simulink library "MinSegLibrary_M2V5"  (R2015a)
settings: Solver=ode45  StartTime=0.0  StopTime=10.0  RelTol=1e-3
libraries: arduinolib x8
settings Model: Creator=hurstj  LastModifiedBy=hurstj
settings DebuggingCC: UnderspecifiedInitializationDetection=Classic  MergeDetectMultiDrivingBlocksExec=none  SolverPrmCheckMsg=warning  StateNameClashWarn=warning

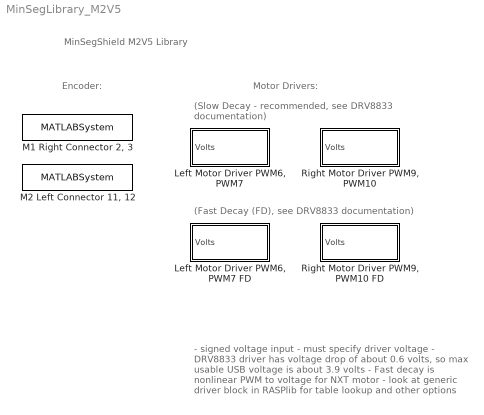
== system MinSegLibrary_M2V5 ==
  note: Encoder:
  note: MinSegShield M2V5 Library
  note: (Slow Decay - recommended, see DRV8833 documentation)
  note: Motor Drivers:
  note: (Fast Decay (FD), see DRV8833 documentation)
  note: - signed voltage input
      | - must specify driver voltage
      | - DRV8833 driver has voltage drop of about 0.6 volts, so max usable USB voltage is about 3.9 volts
      | - Fast decay is nonlinear PWM to voltage for NXT motor
      | - look at generic driver block in RASPlib for table lookup and other options
  "Left Motor Driver PWM6, PWM7" : Subsystem  mask{Vsupply=3.9, PWMoffset=0}
      mask prompts: Vsupply "Driver Voltage"; PWMoffset "PWM offset (0-255)"
      mask help:
      | Specify driver supply voltage (3.9 for USB)
      | Specify the PWM offset (0-255)
      mask Display:
      | port_label('input',1,'Volts')
      | text(15,5,['Vsupply=' num2str(Vsupply)])
  "Left Motor Driver PWM6, PWM7 FD" : Subsystem  mask{Vsupply=3.9, PWMoffset=0}
      mask prompts: Vsupply "Driver Voltage"; PWMoffset "PWM offset (0-255)"
      mask help:
      | Specify driver supply voltage (3.9 for USB)
      | Specify the PWM offset (0-255)
      mask Display:
      | port_label('input',1,'Volts')
      | text(15,5,['Vsupply=' num2str(Vsupply)])
  "M1 Right Connector 2, 3" : MATLABSystem  System=Encoder_arduino  Encoder=0  PinA=2  PinB=3
      mask Type: Encoder_arduino
      mask Display:
      | disp('soEncoder');
      | port_label('output',1,'y');
  "M2 Left Connector 11, 12" : MATLABSystem  System=Encoder_arduino  Encoder=4  PinA=11  PinB=12
      mask Type: Encoder_arduino
      mask Display:
      | disp('soEncoder');
      | port_label('output',1,'y');
  "Right Motor Driver PWM9, PWM10 " : Subsystem  mask{Vsupply=3.9, PWMoffset=0}
      mask prompts: Vsupply "Driver Voltage"; PWMoffset "PWM offset (0-255)"
      mask help:
      | Specify driver supply voltage (3.9 for USB)
      | Specify the PWM offset (0-255)
      mask Display:
      | port_label('input',1,'Volts')
      | text(15,5,['Vsupply=' num2str(Vsupply)])
  "Right Motor Driver PWM9, PWM10 FD" : Subsystem  mask{Vsupply=3.9, PWMoffset=0}
      mask prompts: Vsupply "Driver Voltage"; PWMoffset "PWM offset (0-255)"
      mask help:
      | Specify driver supply voltage (3.9 for USB)
      | Specify the PWM offset (0-255)
      mask Display:
      | port_label('input',1,'Volts')
      | text(15,5,['Vsupply=' num2str(Vsupply)])

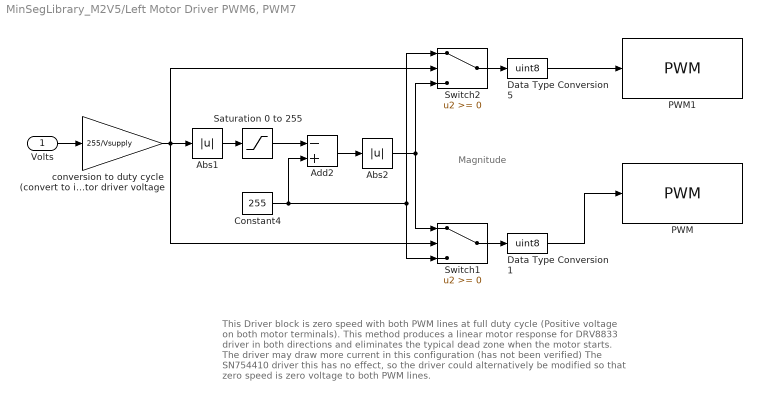
== system MinSegLibrary_M2V5/Left Motor Driver PWM6, PWM7 ==
  note: This Driver block is zero speed with both PWM lines at full duty cycle
      |  (Positive voltage on both motor terminals).
      | This method produces a linear motor response for DRV8833 driver
      |  in both directions and eliminates
      | the typical dead zone when the motor starts.
      | The driver may draw more current in this configuration (has not been verified)
      |
      | The SN754410 driver this has no effect, so the driver could alternatively
      | be modified so that zero speed is zero voltage to both PWM lines.
  note: Magnitude
  Volts : Inport
  Abs1 : Abs
  Abs2 : Abs
  Add2 : Sum  Inputs=-+
  Constant4 : Constant  Value=255
  Data Type Conversion1 : DataTypeConversion  OutDataTypeStr=uint8
  Data Type Conversion5 : DataTypeConversion  OutDataTypeStr=uint8
  PWM : arduinolib/PWM  pinNumber=7  blockPlatform=arduino
  PWM1 : arduinolib/PWM  pinNumber=6  blockPlatform=arduino
  Saturation 0 to 255 : Saturate  UpperLimit=255  LowerLimit=0
  Switch1 : Switch
  Switch2 : Switch
  conversion to duty cycle (convert to int) denominator is motor driver voltage : Gain  Gain=255/Vsupply  OutDataTypeStr=int16
  wires:
  Volts/1 -> conversion to duty cycle (convert to int) denominator is motor driver voltage/1
  conversion to duty cycle (convert to int) denominator is motor driver voltage/1 -> Switch2/2, Abs1/1, Switch1/2
  Saturation 0 to 255/1 -> Add2/1
  Abs1/1 -> Saturation 0 to 255/1
  Constant4/1 -> Switch1/3, Switch2/1, Add2/2
  Add2/1 -> Abs2/1
  Abs2/1 -> Switch2/3, Switch1/1
  Switch2/1 -> Data Type Conversion5/1
  Switch1/1 -> Data Type Conversion1/1
  Data Type Conversion5/1 -> PWM1/1
  Data Type Conversion1/1 -> PWM/1

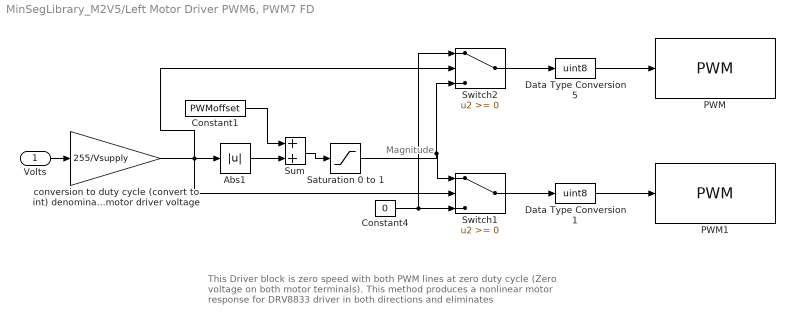
== system MinSegLibrary_M2V5/Left Motor Driver PWM6, PWM7 FD ==
  note: This Driver block is zero speed with both PWM lines at zero duty cycle
      |  (Zero voltage on both motor terminals).
      | This method produces a nonlinear motor response for DRV8833 driver
      |  in both directions and eliminates
  note: Magnitude
  Volts : Inport
  Abs1 : Abs
  Constant1 : Constant  Value=PWMoffset
  Constant4 : Constant  Value=0
  Data Type Conversion1 : DataTypeConversion  OutDataTypeStr=uint8
  Data Type Conversion5 : DataTypeConversion  OutDataTypeStr=uint8
  PWM : arduinolib/PWM  pinNumber=6  blockPlatform=arduino
  PWM1 : arduinolib/PWM  pinNumber=7  blockPlatform=arduino
  Saturation 0 to 1 : Saturate  UpperLimit=255  LowerLimit=0
  Sum : Sum
  Switch1 : Switch
  Switch2 : Switch
  conversion to duty cycle (convert to int) denominator is motor driver voltage : Gain  Gain=255/Vsupply  OutDataTypeStr=int16
  wires:
  Volts/1 -> conversion to duty cycle (convert to int) denominator is motor driver voltage/1
  conversion to duty cycle (convert to int) denominator is motor driver voltage/1 -> Switch1/2, Abs1/1, Switch2/2
  Constant4/1 -> Switch2/1, Switch1/3
  Saturation 0 to 1/1 -> Switch2/3, Switch1/1
  Switch2/1 -> Data Type Conversion5/1
  Switch1/1 -> Data Type Conversion1/1
  Data Type Conversion5/1 -> PWM/1
  Data Type Conversion1/1 -> PWM1/1
  Abs1/1 -> Sum/2
  Sum/1 -> Saturation 0 to 1/1
  Constant1/1 -> Sum/1

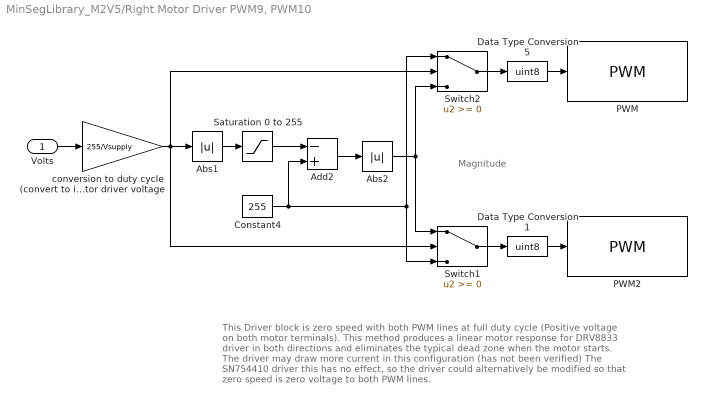
== system MinSegLibrary_M2V5/Right Motor Driver PWM9, PWM10  ==
  note: This Driver block is zero speed with both PWM lines at full duty cycle
      |  (Positive voltage on both motor terminals).
      | This method produces a linear motor response for DRV8833 driver
      |  in both directions and eliminates
      | the typical dead zone when the motor starts.
      | The driver may draw more current in this configuration (has not been verified)
      |
      | The SN754410 driver this has no effect, so the driver could alternatively
      | be modified so that zero speed is zero voltage to both PWM lines.
  note: Magnitude
  Volts : Inport
  Abs1 : Abs
  Abs2 : Abs
  Add2 : Sum  Inputs=-+
  Constant4 : Constant  Value=255
  Data Type Conversion1 : DataTypeConversion  OutDataTypeStr=uint8
  Data Type Conversion5 : DataTypeConversion  OutDataTypeStr=uint8
  PWM : arduinolib/PWM  pinNumber=9  blockPlatform=arduino
  PWM2 : arduinolib/PWM  pinNumber=10  blockPlatform=arduino
  Saturation 0 to 255 : Saturate  UpperLimit=255  LowerLimit=0
  Switch1 : Switch
  Switch2 : Switch
  conversion to duty cycle (convert to int) denominator is motor driver voltage : Gain  Gain=255/Vsupply  OutDataTypeStr=int16
  wires:
  Volts/1 -> conversion to duty cycle (convert to int) denominator is motor driver voltage/1
  conversion to duty cycle (convert to int) denominator is motor driver voltage/1 -> Abs1/1, Switch2/2, Switch1/2
  Saturation 0 to 255/1 -> Add2/1
  Abs1/1 -> Saturation 0 to 255/1
  Constant4/1 -> Switch1/3, Switch2/1, Add2/2
  Add2/1 -> Abs2/1
  Abs2/1 -> Switch2/3, Switch1/1
  Switch2/1 -> Data Type Conversion5/1
  Switch1/1 -> Data Type Conversion1/1
  Data Type Conversion5/1 -> PWM/1
  Data Type Conversion1/1 -> PWM2/1

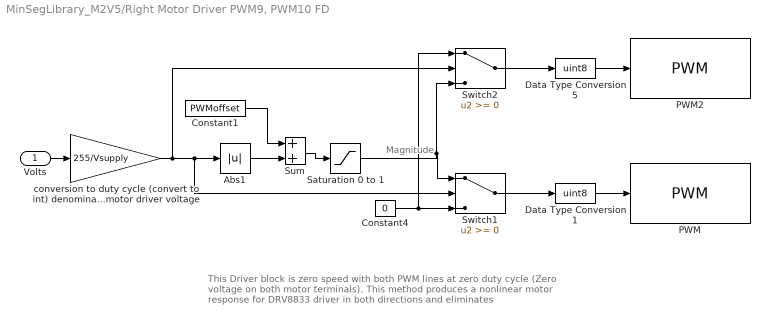
== system MinSegLibrary_M2V5/Right Motor Driver PWM9, PWM10 FD ==
  note: This Driver block is zero speed with both PWM lines at zero duty cycle
      |  (Zero voltage on both motor terminals).
      | This method produces a nonlinear motor response for DRV8833 driver
      |  in both directions and eliminates
  note: Magnitude
  Volts : Inport
  Abs1 : Abs
  Constant1 : Constant  Value=PWMoffset
  Constant4 : Constant  Value=0
  Data Type Conversion1 : DataTypeConversion  OutDataTypeStr=uint8
  Data Type Conversion5 : DataTypeConversion  OutDataTypeStr=uint8
  PWM : arduinolib/PWM  pinNumber=10  blockPlatform=arduino
  PWM2 : arduinolib/PWM  pinNumber=9  blockPlatform=arduino
  Saturation 0 to 1 : Saturate  UpperLimit=255  LowerLimit=0
  Sum : Sum
  Switch1 : Switch
  Switch2 : Switch
  conversion to duty cycle (convert to int) denominator is motor driver voltage : Gain  Gain=255/Vsupply  OutDataTypeStr=int16
  wires:
  Volts/1 -> conversion to duty cycle (convert to int) denominator is motor driver voltage/1
  conversion to duty cycle (convert to int) denominator is motor driver voltage/1 -> Switch1/2, Abs1/1, Switch2/2
  Constant4/1 -> Switch2/1, Switch1/3
  Saturation 0 to 1/1 -> Switch2/3, Switch1/1
  Switch2/1 -> Data Type Conversion5/1
  Switch1/1 -> Data Type Conversion1/1
  Data Type Conversion5/1 -> PWM2/1
  Data Type Conversion1/1 -> PWM/1
  Abs1/1 -> Sum/2
  Sum/1 -> Saturation 0 to 1/1
  Constant1/1 -> Sum/1
